simulink model "test_test_sys_characteristics"  (R2019a)
settings: Solver=FixedStepAuto  StartTime=0.0  StopTime=Tend  FixedStep=ts  RelTol=1e-3
values from neighbouring files (symbols this model uses):
  den = [1 1]    [tset_1.m]
  num = [1]    [tset_1.m]
  Tend = 40    [tset_1.m]
  w1 = fmax*2*pi    (= 0.948760981384)    [tset_1.m]
libraries: simulink x1
settings Model: Creator=lzr96  LastModifiedBy=lzr96

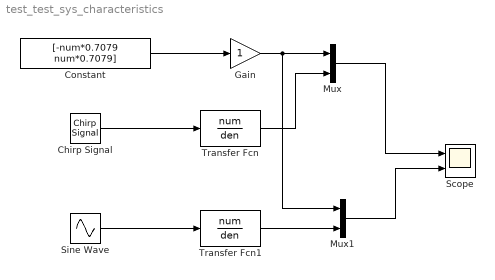
== system test_test_sys_characteristics ==
  Chirp Signal : simulink/Sources/Chirp Signal  f1=Fstart  T=Tend  f2=Fend
  Constant : Constant  Value=[-num*0.7079 num*0.7079]
  Gain : Gain
  Mux : Mux  Inputs=2
  Mux1 : Mux  Inputs=2
  Scope : Scope  NumInputPorts=2
  Sine Wave : Sin  Frequency=w1  SampleTime=0
  Transfer Fcn : TransferFcn  Numerator=num  Denominator=den
  Transfer Fcn1 : TransferFcn  Numerator=num  Denominator=den
  wires:
  Chirp Signal/1 -> Transfer Fcn/1
  Sine Wave/1 -> Transfer Fcn1/1
  Constant/1 -> Gain/1
  Gain/1 -> Mux1/1, Mux/1
  Transfer Fcn/1 -> Mux/2
  Transfer Fcn1/1 -> Mux1/2
  Mux/1 -> Scope/1
  Mux1/1 -> Scope/2
